simulink model "NewtonMRAC"  (R2022b)
settings: Solver=ode4  StartTime=0.0  StopTime=50  FixedStep=1e-3  RelTol=1e-5  AbsTol=1e-7
values from neighbouring files (symbols this model uses):
  A = -1    [UniCenterMRAC.m]    (also in createPoints.m = []; greedySet2.m = []; runCompareBasisMRAC.m; runNewtonMRAC.m = -4)
  alpha0 = 0    [Run_Both_Model.m]    (also in Run_Deadzone.m; Run_ScalarModel.m; Slicing.m; UniCenterMRAC.m)
  Ar = -1    [UniCenterMRAC.m]    (also in runCompareBasisMRAC.m; runNewtonMRAC.m = -5; runTriggerTest.m = -10000; runVanDerPolTrigger.m = A)
  B = 1    [UniCenterMRAC.m]    (also in cholNP.m = A(kk:n,kk:n); cholwPiv.m = A(kk:n,kk:n); pivchol.m = A(kk:n,kk:n); runCompareBasisMRAC.m)
  beta0 = 0    [Run_Both_Model.m]    (also in Run_Deadzone.m; Run_ScalarModel.m; Slicing.m; UniCenterMRAC.m)
  Br = 1    [UniCenterMRAC.m]    (also in runCompareBasisMRAC.m; runNewtonMRAC.m; runTriggerTest.m; runVanDerPolTrigger.m = B)
  centers = linspace(-OmegaLim-ext,OmegaLim+ext,N)'    [UniCenterMRAC.m]    (also in getOfflineError.m = linspace(-OmegaLim-ext,OmegaLim+ext,Ns(nn))'; getOfflineErrorNewt.m = linspace(-OmegaLim-ext,OmegaLim+ext,Ns(nn))'; getOfflineErrorNewt2.m = linspace(-OmegaLim-ext,OmegaLim+ext,Ns(nn))'; getVDP_HNorm.m = omegaCover2(Ri,Ro,h(hh)))
  Dim = 1    [UniCenterMRAC.m]    (also in runCompareBasisMRAC.m; runNewtonMRAC.m; runTriggerTest.m; runWendlandMRAC.m)
  epsilon = powBound(nn)*norm_fs+delta    [UniCenterMRAC.m]    (also in runCompareBasisMRAC.m; runNewtonMRAC.m; runTriggerTest.m = PowerBound+delta; runVanDerPolTrigger.m = PowerBound*R+delta)
  ga = 10    [Run_Both_Model.m]    (also in Run_Deadzone.m; Run_ScalarModel.m; Slicing.m; UniCenterMRAC.m = 0)
  gb = 10    [Run_Both_Model.m]    (also in Run_Deadzone.m; Run_ScalarModel.m; Slicing.m; UniCenterMRAC.m = 0)
  gf = 10    [Run_Both_Model.m]    (also in Run_Deadzone.m; Run_ScalarModel.m; Slicing.m; UniCenterMRAC.m = 1)
  interps = linspace(-OmegaLim,OmegaLim,Ip)'    [UniCenterMRAC.m]    (also in runCompareBasisMRAC.m; runNewtonMRAC.m; runTriggerTest.m; runWendlandMRAC.m)
  norm_fs = max(norm_fs)    [createPoints.m]    (also in getOfflineError.m = max(norm_fs(condNum < 10^5)); getOfflineErrorNewt.m = max(norm_fsStand(condNum < 10^5)); getOfflineErrorNewt2.m = max(norm_fs(condNum < 10^5)); greedyCenters.m)
  par = 1    [UniCenterMRAC.m]    (also in frbf.m = par-2; runCompareBasisMRAC.m; runNewtonMRAC.m; runTriggerTest.m)
  scale = 0.2    [UniCenterMRAC.m]    (also in runCompareBasisMRAC.m = 0.1; runNewtonMRAC.m = 0.5; runTriggerTest.m = 0.1; runVanDerPolTrigger.m = 0.3)
  sigma = 0.1    [Run_Both_Model.m]    (also in Run_Deadzone.m; Run_Project1i_haoran9.m; Run_ScalarModel.m; Slicing.m)
  SNU = 10    [UniCenterMRAC.m]    (also in runCompareBasisMRAC.m = 2; runNewtonMRAC.m; runTriggerTest.m = 2; runWendlandMRAC.m)
  StartMeasureTime = runTimes(tt)-1    [UniCenterMRAC.m]    (also in runCompareBasisMRAC.m = runTimes(tt)-10; runNewtonMRAC.m = runTimes(tt)-10; runTriggerTest.m = 0; runVanDerPolTrigger.m = 1990)
  targetCoefs = intmat\ySamps    [UniCenterMRAC.m]    (also in runCompareBasisMRAC.m; runNewtonMRAC.m; runTriggerTest.m; runWendlandMRAC.m)
  targetNu = 1/2*(sTarget+Dim/2)    (= 1.75)    [UniCenterMRAC.m]    (also in runCompareBasisMRAC.m; runNewtonMRAC.m; runTriggerTest.m; runWendlandMRAC.m)
  targetScale = 0.2    [UniCenterMRAC.m]    (also in runCompareBasisMRAC.m; runNewtonMRAC.m; runTriggerTest.m; runWendlandMRAC.m)
  x0 = 0    [Run_Both_Model.m]    (also in Run_Deadzone.m; Run_Project1i_haoran9.m = 1; Run_ScalarModel.m; Slicing.m = 5)
  xr0 = 0    [Run_Both_Model.m]    (also in Run_Deadzone.m; Run_Project1i_haoran9.m; Run_ScalarModel.m; Slicing.m)
libraries: simulink x4
settings Model: Creator=owned  LastModifiedBy=Nathan
settings SolverCC: AlgebraicLoopSolver=TrustRegion
settings DebuggingCC: UnderSpecifiedDataTypeMsg=warning  UnconnectedInputMsg=warning  UnconnectedOutputMsg=warning  UnconnectedLineMsg=warning  SFMachineParentedDataDiag=warning  UnderSpecifiedDimensionMsg=warning
settings ModelReferenceCC: EnableRefExpFcnMdlSchedulingChecks=on
settings RTWCC: DLArmComputeVersion=19.05

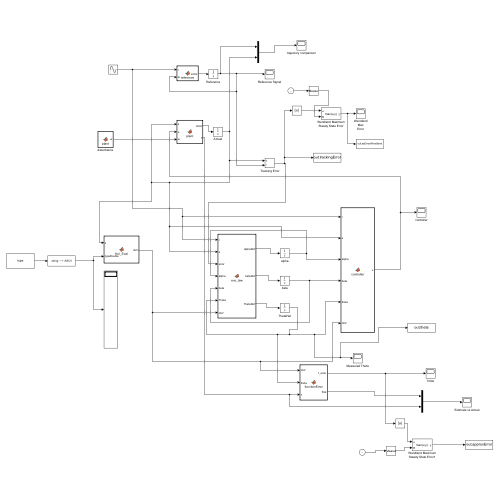
[thumbnail: Simulink's stored preview of the top-level diagram]
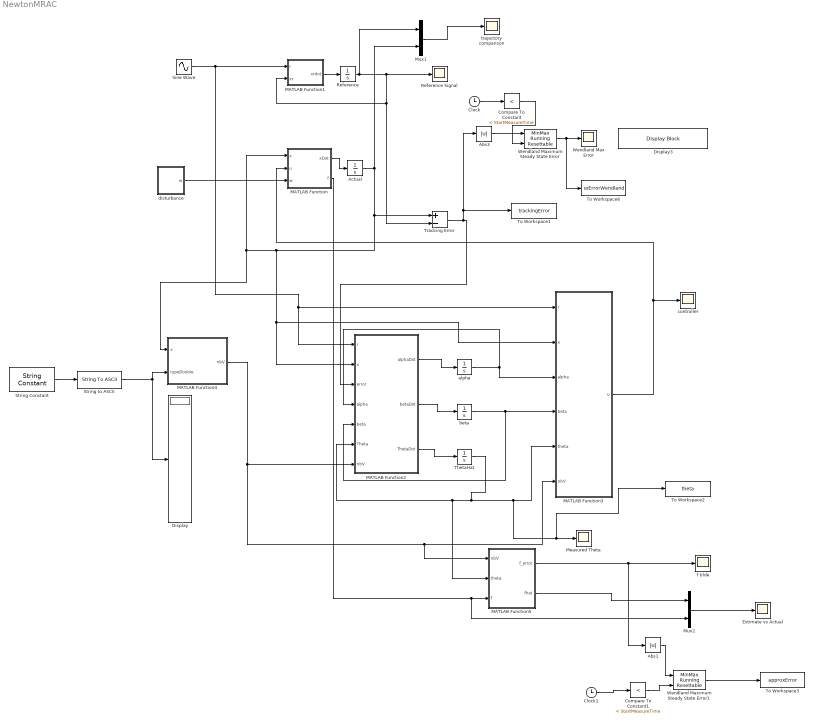
== system NewtonMRAC ==
  " Tracking Error" : Sum  Inputs=+-
  Abs1 : Abs  SaturateOnIntegerOverflow=off
  Abs3 : Abs  SaturateOnIntegerOverflow=off
  Actual : Integrator  InitialCondition=x0
  Clock : Clock
  Clock1 : Clock
  Compare To Constant : simulink/Logic and Bit Operations/Compare To Constant  relop=<  const=StartMeasureTime  OutDataTypeStr=boolean
  Compare To Constant1 : simulink/Logic and Bit Operations/Compare To Constant  relop=<  const=StartMeasureTime  OutDataTypeStr=boolean
  Display : Display
  Display3 : DisplayBlock  LabelPosition=Hide  Transparency=1
  Estimate vs Actual : Scope
  MATLAB Function : MATLAB Function  TreatAsAtomicUnit=on
  MATLAB Function1 : MATLAB Function  TreatAsAtomicUnit=on
  MATLAB Function2 : MATLAB Function  TreatAsAtomicUnit=on
  MATLAB Function3 : MATLAB Function  TreatAsAtomicUnit=on
  MATLAB Function4 : MATLAB Function  TreatAsAtomicUnit=on
  MATLAB Function5 : MATLAB Function  TreatAsAtomicUnit=on
  Measured Theta : Scope
  Mux1 : Mux  Inputs=2
  Mux2 : Mux  Inputs=2
  Reference : Integrator  InitialCondition=xr0
  Reference Signal : Scope
  Sine Wave : Sin  Amplitude=norm_fs*SNU  Frequency=2*pi  SampleTime=0
  String Constant : StringConstant  String=type
  String to ASCII : StringToASCII
  ThetaHat : Integrator
  To Workspace1 : ToWorkspace  VariableName=trackingError  SaveFormat=Timeseries  SampleTime=-1
  To Workspace2 : ToWorkspace  VariableName=theta  SaveFormat=Timeseries  SampleTime=-1
  To Workspace3 : ToWorkspace  VariableName=approxError  SaveFormat=Timeseries  SampleTime=-1
  To Workspace6 : ToWorkspace  VariableName=ssErrorWendland  SaveFormat=Timeseries  SampleTime=-1
  Wendland Max Error : Scope
  Wendland Maximum Steady State Error : simulink/Math Operations/MinMax Running Resettable  Function=max  vinit=0.0
  Wendland Maximum Steady State Error1 : simulink/Math Operations/MinMax Running Resettable  Function=max  vinit=0.0
  alpha : Integrator  InitialCondition=alpha0
  beta : Integrator  InitialCondition=beta0
  controller : Scope
  disturbance : MATLAB Function  TreatAsAtomicUnit=on
  f tilde : Scope
  trajectory comparison : Scope
  wires:
  Sine Wave/1 -> MATLAB Function1/1(r), MATLAB Function2/1(r), MATLAB Function3/1(r)
  MATLAB Function1/1(xrdot) -> Reference/1
  Reference/1 -> " Tracking Error"/2, MATLAB Function1/2(xr), Reference Signal/1, Mux1/1
  MATLAB Function/1(xDot) -> Actual/1
  Actual/1 -> " Tracking Error"/1, MATLAB Function/1(x), MATLAB Function4/1(x), MATLAB Function2/2(x), MATLAB Function3/2(x), Mux1/2
  " Tracking Error"/1 -> MATLAB Function2/3(error), Abs3/1, To Workspace1/1
  MATLAB Function2/1(alphaDot) -> alpha/1
  MATLAB Function2/2(betaDot) -> beta/1
  MATLAB Function2/3(ThetaDot) -> ThetaHat/1
  MATLAB Function4/1(nbV) -> MATLAB Function5/1(nbV), MATLAB Function3/6(nbV), MATLAB Function2/7(nbV)
  alpha/1 -> MATLAB Function3/3(alpha), MATLAB Function2/4(alpha)
  beta/1 -> MATLAB Function2/5(beta), MATLAB Function3/4(beta)
  ThetaHat/1 -> To Workspace2/1, Measured Theta/1, MATLAB Function3/5(theta), MATLAB Function5/2(theta), MATLAB Function2/6(Theta)
  MATLAB Function3/1(u) -> MATLAB Function/2(u), controller/1
  Clock/1 -> Compare To Constant/1
  Compare To Constant/1 -> Wendland Maximum Steady State Error/2
  Wendland Maximum Steady State Error/1 -> To Workspace6/1, Wendland Max Error/1
  Abs3/1 -> Wendland Maximum Steady State Error/1
  Mux1/1 -> trajectory comparison/1
  String Constant/1 -> String to ASCII/1
  String to ASCII/1 -> Display/1, MATLAB Function4/2(typeDouble)
  MATLAB Function/2(f) -> Mux2/2, MATLAB Function5/3(f)
  MATLAB Function5/1(f_error) -> Abs1/1, f tilde/1
  Mux2/1 -> Estimate vs Actual/1
  MATLAB Function5/2(fhat) -> Mux2/1
  Clock1/1 -> Compare To Constant1/1
  Abs1/1 -> Wendland Maximum Steady State Error1/1
  Compare To Constant1/1 -> Wendland Maximum Steady State Error1/2
  Wendland Maximum Steady State Error1/1 -> To Workspace3/1
  disturbance/1(w) -> MATLAB Function/3(w)

== matlab function NewtonMRAC/MATLAB Function3 ==
  data: r input; x input; alpha input; beta input; theta input; nbV input; u output size=1; epsilon parameter; B parameter
function u = controller(r, x,alpha,beta, theta,nbV,epsilon,B)
% P= 1;
% if B*P*x >= 0
%     vN = epsilon;
% else
%     vN = -epsilon;
% end
u = alpha*x+beta*r-theta'*nbV;
end

== matlab function NewtonMRAC/MATLAB Function4 ==
  data: x input; centers parameter; typeDouble input; nbV output; scale parameter; par parameter
function nbV  = Knl_Eval(x,centers, typeDouble, scale, par)
  
    type = char(typeDouble(typeDouble~=0));
    
    N = length(centers);
    V = zeros(N,N);
    knlV = real(kermat(centers,x,type,par,scale));
    
    Z = real(kermat(centers,centers,type,par,scale));
    z = diag(Z);
    
    v_x = zeros(N,1);
    P = sqrt(real(kermat(centers(1),centers(1),type,par,scale)));
    
    v_x(1) = knlV(1)/P;
    
    
    if N > 1
        V(:,1) = real(kermat(centers(1),centers,type,par,scale))/P;
        w = V(:,1).^2;
        NN = V(2,:)*v_x;
        P = sqrt(z(2)-w(2));
        
        for jj = 1:N-1
            e = zeros(N,1);
            e(jj+1) = 1;
            Vm = V(:,1:jj);
            u = real(kermat(centers,centers(jj+1),type,par,scale))-Vm*Vm'*e;
            u_x = knlV(jj+1) - NN;
            v_x(jj+1) = u_x/P; % Newton Basis evaluated at x
            V(:,jj+1) = u/P; % Newton Basis evaluated at the centers
            w = V(:,jj+1).^2 + w; % Updating sum of Newton basis squared at the centers
            if jj ~=N-1
                NN = V(jj+2,:)*v_x;
                P = sqrt(z(jj+2)-w(jj+2));
            end
        end
    end
    nbV = v_x;
end

== matlab function NewtonMRAC/MATLAB Function5 ==
  data: nbV input; f_error output size=1; theta input; f input; fhat output
function [f_error,fhat]  = functionError(nbV,theta, f)
fhat = theta'*nbV;
f_error = f-fhat;

== matlab function NewtonMRAC/disturbance ==
  data: w output; delta parameter
function w   = plant(delta)
% 
w = 0.5*rand;

== matlab function NewtonMRAC/MATLAB Function1 ==
  data: r input; xr input; xrdot output; Ar parameter; Br parameter
function xrdot = reference(r,xr,Ar, Br)

xrdot = Ar*xr+Br*r;

== matlab function NewtonMRAC/MATLAB Function ==
  data: x input; u input; A parameter; B parameter; w input; interps parameter; targetCoefs parameter; xDot output; f output; targetScale parameter; targetNu parameter; Dim parameter
function [xDot,f]  = plant(x,u,A, B,w,interps, targetCoefs,targetScale,targetNu, Dim)
% 
targetKnlV = real(kermat(interps,x,'ms',targetNu-Dim/2,targetScale));
f = targetCoefs'*targetKnlV;


xDot = A*x+B*(u+f+w);

== matlab function NewtonMRAC/MATLAB Function2 ==
  data: ga parameter; gb parameter; gf parameter; sigma parameter; alphaDot output size=1; betaDot output size=1; ThetaDot output size=N; r input; x input; error input; alpha input; beta input; Theta input; nbV input; epsilon parameter
function [alphaDot, betaDot, ThetaDot] = evo_law(ga, gb, gf, sigma, r, x, error, alpha, beta, Theta, nbV, epsilon)


%% Standard RKHS Sigma Mod
% alphaDot=-ga*x*error-sigma*alpha;
% betaDot=-gb*r*error-sigma*beta;
% ThetaDot=gf*invK*knlV*error-sigma*Theta;

%% Standard RKHS Deadzone
if abs(error) > epsilon
    alphaDot=-ga*x*error;
    betaDot=-gb*r*error;
    ThetaDot=gf*nbV*error;
else
    alphaDot=0;
    betaDot=0;
    ThetaDot=zeros(size(nbV));
end


%% Standard RKHS Deadzone
% if abs(error)>epsilon
%     alphaDot=-ga*x*error;
%     betaDot=-gb*r*error;
%     ThetaDot=gf*K\knlV*error;
% else
%     alphaDot=0;
%     betaDot=0;
%     ThetaDot=zeros(size(knlV));
% end
